simulink model "cPIDMF"  (R2018a)
settings: Solver=VariableStepAuto  StartTime=0.0  StopTime=3.0  RelTol=1e-3
libraries: simulink x1
settings Model: Creator=robotica  LastModifiedBy=JMONTIELG
settings CodeAppCC: StateflowObjectComments=on

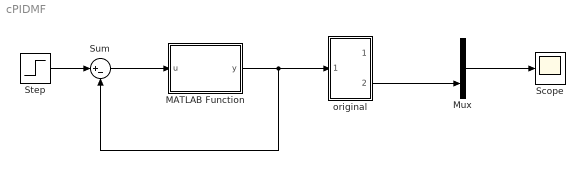
== system cPIDMF ==
  MATLAB Function : MATLAB Function  TreatAsAtomicUnit=on
  Mux : Mux  Inputs=2
  Scope : Scope
  Step : Step  SampleTime=1
  Sum : Sum  Inputs=|+-
  original : Subsystem
  wires:
  Mux/1 -> Scope/1
  original/2(clean) -> Mux/2
  MATLAB Function/1(y) -> Sum/2, original/1(signal)
  Step/1 -> Sum/1
  Sum/1 -> MATLAB Function/1(u)

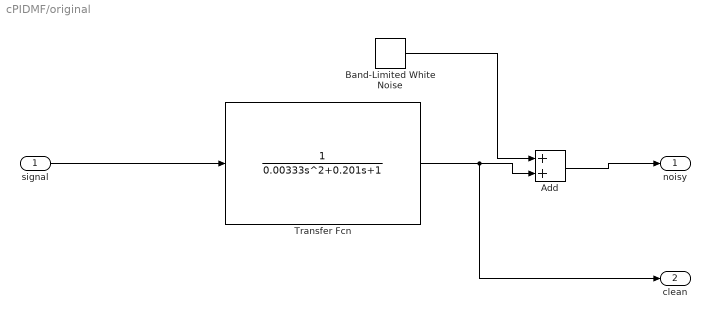
== system cPIDMF/original ==
  signal : Inport
  Add : Sum
  Band-Limited White Noise : simulink/Sources/Band-Limited White Noise  Cov=[0.0000001]  Ts=0.001  seed=[23341]
  Transfer Fcn : TransferFcn  Denominator=[0.00333 0.201 1]
  noisy : Outport
  clean : Outport  Port=2
  wires:
  Transfer Fcn/1 -> clean/1, Add/2
  Band-Limited White Noise/1 -> Add/1
  Add/1 -> noisy/1
  signal/1 -> Transfer Fcn/1

== matlab function cPIDMF/MATLAB Function ==
  data: u input; y output
function y = fcn(u)
Kp=45.45;
Ki=31.4141;
Kd=0;
p=Kp*u;
i=Ki*u^2/2;
d=Kd*u;

u=p+i+d;
y = u;
